simulink model "diff_eqn"  (R2017a)
settings: Solver=VariableStepAuto  StartTime=0.0  StopTime=10.0  RelTol=1e-3
settings Model: Creator=Bob  LastModifiedBy=Bob

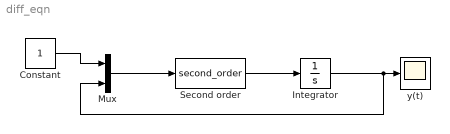
== system diff_eqn ==
  Constant : Constant
  Integrator : Integrator  InitialCondition=0.5
  Mux : Mux  Inputs=2
  Second order : MATLABFcn  MATLABFcn=second_order  OutputDimensions=2
  y(t) : Scope
  wires:
  Second order/1 -> Integrator/1
  Integrator/1 -> Mux/2, y(t)/1
  Mux/1 -> Second order/1
  Constant/1 -> Mux/1
